simulink model "Cruise_Control_Referenced"  (R2020b)
settings: Solver=ode45  StartTime=0.0  StopTime=10  RelTol=1e-3
values from neighbouring files (symbols this model uses):
  b = 50.0    [Dictionary.sldd]
  m = 1000.0    [Dictionary.sldd]
settings Model: DataDictionary=Dictionary.sldd  Creator=abhin  LastModifiedBy=abhin
settings DataIOCC: SaveOutput=off  SaveTime=off

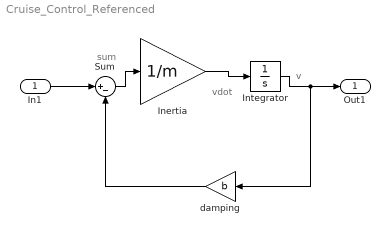
== system Cruise_Control_Referenced ==
  note: vdot
  note: sum
  note: v
  In1 : Inport  OutDataTypeStr=double  PortDimensions=1  SampleTime=0
  Inertia : Gain  Gain=1/m
  Integrator : Integrator
  Sum : Sum  Inputs=|+-
  damping : Gain  Gain=b
  Out1 : Outport  OutDataTypeStr=double  PortDimensions=1  SampleTime=0
  wires:
  In1/1 -> Sum/1
  Sum/1 -> Inertia/1
  Inertia/1 -> Integrator/1
  damping/1 -> Sum/2
  Integrator/1 -> damping/1, Out1/1
